simulink model "MatLab1com"  (Simulink 7.1)
settings: Solver=ode45  StartTime=0.0  StopTime=10000  FixedStep=0.001  RelTol=1e-3
settings Model: Creator=Denise e Hector  LastModifiedBy=hector
settings DebuggingCC: SaveWithParameterizedLinksMsg=none
settings GRTTargetCC: TargetFcnLib=ansi_tfl_tmw.mat

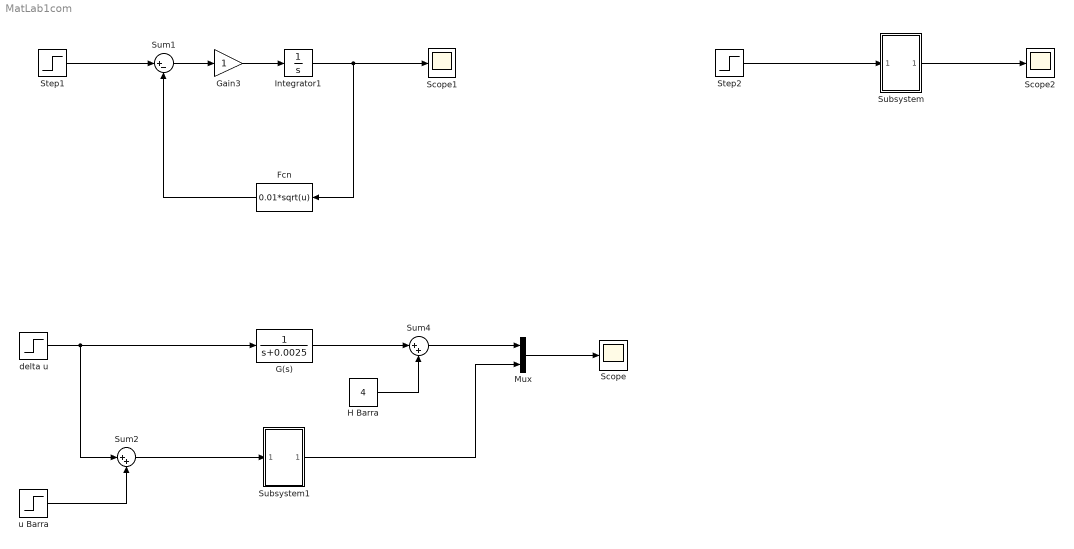
== system MatLab1com ==
  Fcn : Fcn  Orientation=left  Expr=0.01*sqrt(u)
  G(s) : TransferFcn  Denominator=[1 0.0025]
  Gain3 : Gain  ParameterDataType=sfix(16)  ParameterScaling=2^0  OutDataType=sfix(16)  OutScaling=2^0
  H Barra : Constant  Value=4  OutDataType=sfix(16)  OutScaling=2^0
  Integrator1 : Integrator
  Mux : Mux  Inputs=2
  Scope : Scope
      settings: YMin=3.999  YMax=4.00175
  Scope1 : Scope
      settings: YMin=3.6125  YMax=3.66
  Scope2 : Scope
      settings: YMin=3.6125  YMax=3.66  SaveName=ScopeData4
  Step1 : Step  Time=0  After=0.1  SampleTime=0
  Step2 : Step  Time=0  After=0.1  SampleTime=0
  Subsystem : Subsystem
  Subsystem1 : Subsystem
  Sum1 : Sum  Inputs=|+-  OutDataType=sfix(16)  OutScaling=2^0
  Sum2 : Sum  Inputs=|++  OutDataType=sfix(16)  OutScaling=2^0
  Sum4 : Sum  Inputs=|++  OutDataType=sfix(16)  OutScaling=2^0
  delta u : Step  Time=5000  After=0.0001  SampleTime=0
  u Barra : Step  Time=0  After=0.02  SampleTime=0
  wires:
  Step1/1 -> Sum1/1
  Fcn/1 -> Sum1/2
  Integrator1/1 -> Scope1/1, Fcn/1
  Gain3/1 -> Integrator1/1
  Sum1/1 -> Gain3/1
  delta u/1 -> G(s)/1, Sum2/1
  G(s)/1 -> Sum4/1
  Sum4/1 -> Mux/1
  H Barra/1 -> Sum4/2
  Mux/1 -> Scope/1
  Step2/1 -> Subsystem/1(In1)
  Subsystem/1(Out1) -> Scope2/1
  Subsystem1/1(Out1) -> Mux/2
  u Barra/1 -> Sum2/2
  Sum2/1 -> Subsystem1/1(In1)

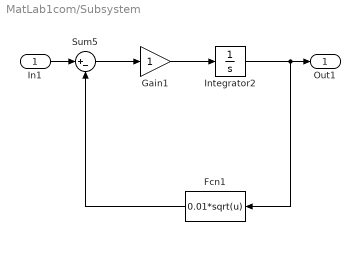
== system MatLab1com/Subsystem ==
  In1 : Inport
  Fcn1 : Fcn  Orientation=left  Expr=0.01*sqrt(u)
  Gain1 : Gain  ParameterDataType=sfix(16)  ParameterScaling=2^0  OutDataType=sfix(16)  OutScaling=2^0
  Integrator2 : Integrator
  Sum5 : Sum  Inputs=|+-  OutDataType=sfix(16)  OutScaling=2^0
  Out1 : Outport
  wires:
  Fcn1/1 -> Sum5/2
  Integrator2/1 -> Fcn1/1, Out1/1
  Gain1/1 -> Integrator2/1
  Sum5/1 -> Gain1/1
  In1/1 -> Sum5/1

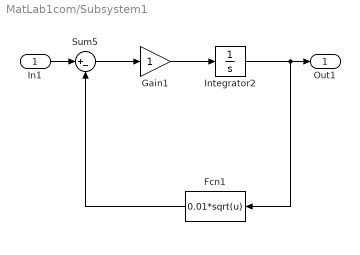
== system MatLab1com/Subsystem1 ==
  In1 : Inport
  Fcn1 : Fcn  Orientation=left  Expr=0.01*sqrt(u)
  Gain1 : Gain  ParameterDataType=sfix(16)  ParameterScaling=2^0  OutDataType=sfix(16)  OutScaling=2^0
  Integrator2 : Integrator
  Sum5 : Sum  Inputs=|+-  OutDataType=sfix(16)  OutScaling=2^0
  Out1 : Outport
  wires:
  Fcn1/1 -> Sum5/2
  Integrator2/1 -> Fcn1/1, Out1/1
  Gain1/1 -> Integrator2/1
  Sum5/1 -> Gain1/1
  In1/1 -> Sum5/1
